simulink subsystem "Automotive_Suspension_6DOF"  (R2024a)
settings: Solver=VariableStepAuto  StartTime=0.0  StopTime=10.0  RelTol=1e-3
libraries: vehdynlibeom x1
settings Model: Creator=USER  LastModifiedBy=USER

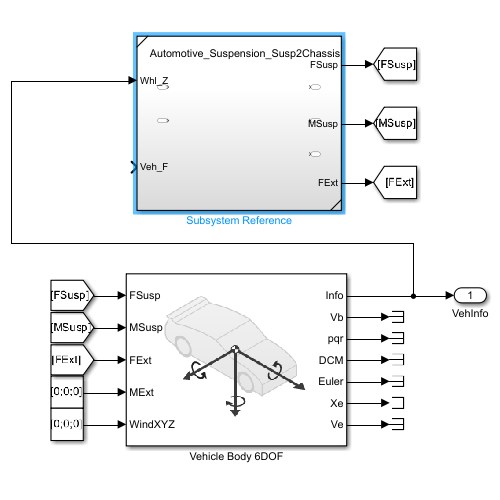
[thumbnail: Simulink's stored preview of the top-level diagram]
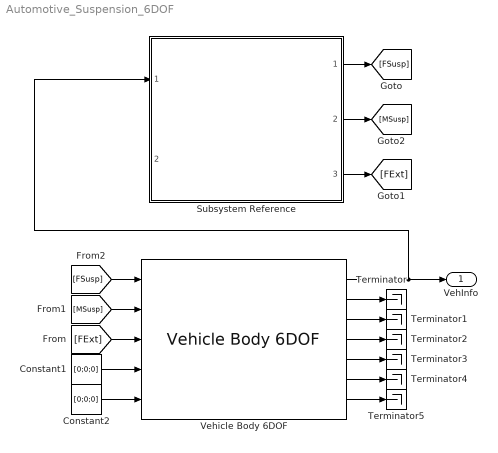
== system Automotive_Suspension_6DOF ==
  Constant1 : Constant  Value=[0;0;0]
  Constant2 : Constant  Value=[0;0;0]
  Subsystem Reference : Subsystem  ReferencedSubsystem=Automotive_Suspension_Susp2Chassis
  Terminator{,1..5} (6 alike) : Terminator
  Vehicle Body 6DOF : vehdynlibeom/Vehicle Body 6DOF  extPos=on  extVel=on  extEuler=on  extRotRate=on  htchFMode=off  htchMMode=off  m=2000  a=1.4  b=1.6  d=0  h=0.35  dh=1  hl=0  hh=0.1  Xe_o=[0,0,0]  xbdot_o=[0,0,0]  eul_o=[0,0,0]  p_o=[0,0,0]  Iveh=[430 0 0; 0 1900 0; 0 0 2100]  w=[1.9,1.9]  z1m=0  z1R=[-.25,.125,.15]  z1I=[1.4,-.2,.1;-.2,1.4,.1;.1,.1,2.25].*0  z2m=0  z2R=[1.4,0,.8]  z2I=[1.4,-.2,.1;-.2,1.4,.1;.1,.1,2.25].*0  z3m=0  z3R=[.75,-.5,.4]  z3I=[5,-.1,-2;-2,9,.1;-.1,.1,6].*0  z4m=0  z4R=[.75,.5,.4]  z4I=[5,-.1,-2;-2,9,.1;-.1,.1,6].*0  z5m=0  z5R=[1.25,-.5,.4]  z5I=[5,-.1,-2;-2,9,.1;-.1,.1,6].*0  z6m=0  z6R=[1.25,-.5,.4]  z6I=[5,-.1,-2;-2,9,.1;-.1,.1,6].*0  z7m=0  z7R=[2,0,.25]  z7I=[1.4,-.2,.1;-.2,1.4,.1;.1,.1,2.25].*0  Af=2  Cd=.3  Cl=.1  Cpm=.1  beta_w=[0:0.001:0.01]  Cs=[0:0.01:0.1]  Cym=[0:0.001:0.01]  Pabs=101325  extTamb=off  Tair=273  g=9.81  xdot_tol=.1  longOff=0  latOff=0  vertOff=0  wrapAng=on  aMode=2
  VehInfo : Outport
  wires:
  Vehicle Body 6DOF/2 -> Terminator/1
  Vehicle Body 6DOF/3 -> Terminator1/1
  Vehicle Body 6DOF/7 -> Terminator5/1
  Vehicle Body 6DOF/6 -> Terminator4/1
  Vehicle Body 6DOF/5 -> Terminator3/1
  Vehicle Body 6DOF/4 -> Terminator2/1
  Vehicle Body 6DOF/1 -> Subsystem Reference/1, VehInfo/1
  Constant1/1 -> Vehicle Body 6DOF/4
  Constant2/1 -> Vehicle Body 6DOF/5
  [FExt] -> Vehicle Body 6DOF/3
  [MSusp] -> Vehicle Body 6DOF/2
  [FSusp] -> Vehicle Body 6DOF/1
  Subsystem Reference/1 -> [FSusp]
  Subsystem Reference/2 -> [MSusp]
  Subsystem Reference/3 -> [FExt]
